simulink model "Week2_Simulation"  (R2024b)
settings: Solver=VariableStepAuto  StartTime=0.0  StopTime=10.0  RelTol=1e-3
undefined symbols (not defined in the file or in its folder): vehicleData
settings Model: Creator=Ian  LastModifiedBy=Ian

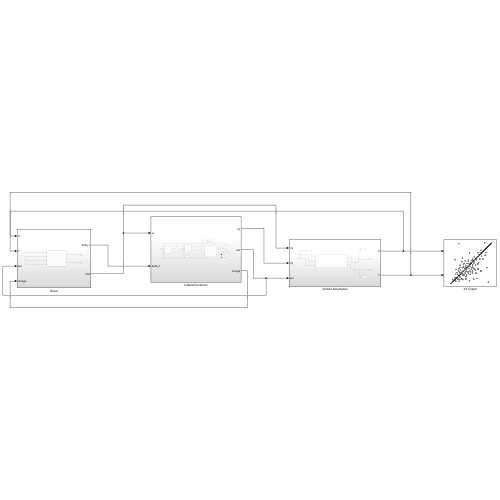
[thumbnail: Simulink's stored preview of the top-level diagram]
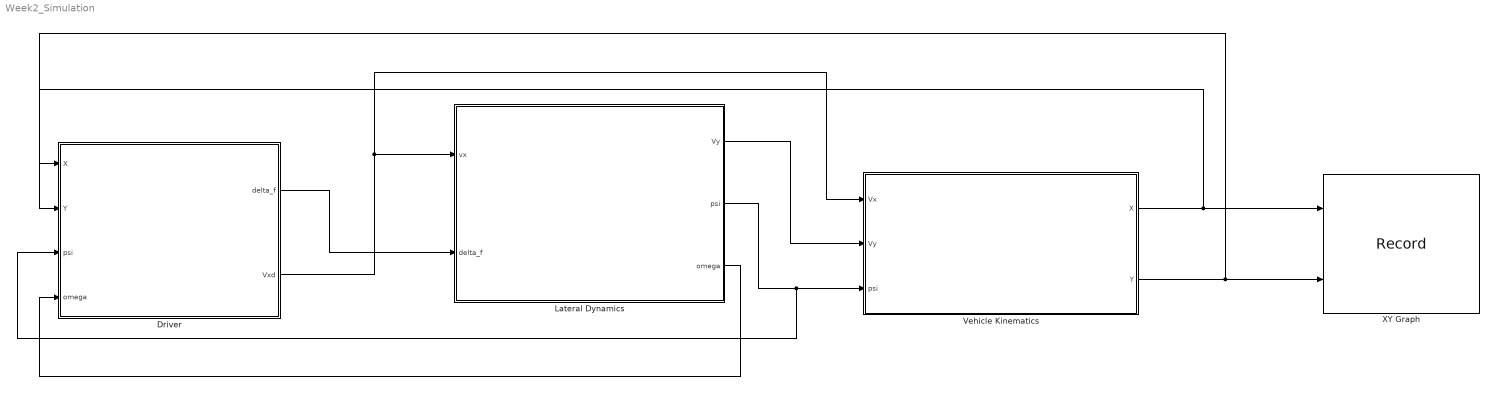
== system Week2_Simulation ==
  Driver : Subsystem
  Lateral Dynamics : Subsystem
  Vehicle Kinematics : Subsystem
  XY Graph : Record  FileSettingsInternal="{\"entries\":[{\"content\":{\"excelSettings\":{\"content\":{},\"type\":\"Streamout.ExcelSettings\"}},\"type\":\"Streamout.FileSettingStorage\",\"uuid\":\"\"}],\"packageUris\":[\"http:\\/\\/schema.mathworks.com\\/mf0\\/streamout_blocks\\/R2020a\"],\"version\":\"1.0\"}"  Layout=[1 1]  SignalsInternal="{\"entries\":[{\"content\":{\"signals\":[{\"content\":{\"blockPath\":[],\"dimensions\":[1],\"domain\":\"\",\"lineColor\":\"#a2142f\",\"plots\":[ 1 ],\"port\":1,\"signalID\":1,\"signalName\":\"XY Graph:1\"},\"type\":\"RecordBlkView.Signal\",\"uuid\":\"\"},{\"content\":{\"blockPath\":[],\"dimensions\":[1],\"domain\":\"\",\"lineColor\":\"#139fff\",\"plots\":[ 1 ],\"port\":2,\"signalID\":2,\"signalName\":\"XY Graph:2\"},\"type\":\"RecordBlkView.Signal\",\"uuid\":\"\"}]},\"type\":\"RecordBlkView.InputSignals\",\"uuid\":\"\"}],\"packageUris\":[\"http:\\/\\/schema.mathworks.com\\/mf0\\/streamout_blocks\\/R2020a\"],\"version\":\"1.0\"}"  VisualizationBindings="{\"xyplotplugin\":{\"info\":[{\"series\":[{\"bindingParametersList\":[{\"parameter\":\"X-Axis\",\"signalID\":1,\"signalName\":\"XY Graph:1\"},{\"parameter\":\"Y-Axis\",\"signalID\":2,\"signalName\":\"XY Graph:2\"}],\"seriesID\":0}],\"subplotID\":1}]}}"  CompatibilityTag=XY
  wires:
  Vehicle Kinematics/2(Y) -> Driver/2(Y), XY Graph/2
  Driver/1(delta_f) -> Lateral Dynamics/2(delta_f)
  Driver/2(Vxd) -> Vehicle Kinematics/1(Vx), Lateral Dynamics/1(vx)
  Vehicle Kinematics/1(X) -> Driver/1(X), XY Graph/1
  Lateral Dynamics/2(psi) -> Driver/3(psi), Vehicle Kinematics/3(psi)
  Lateral Dynamics/1(Vy) -> Vehicle Kinematics/2(Vy)
  Lateral Dynamics/3(omega) -> Driver/4(omega)

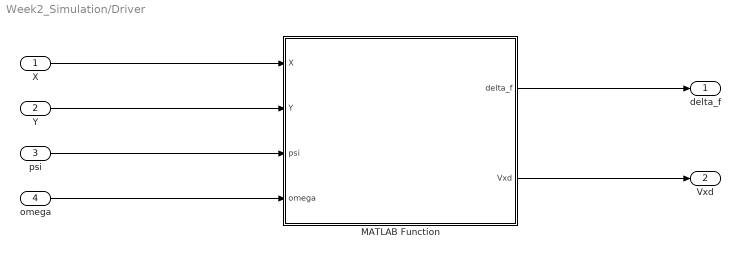
== system Week2_Simulation/Driver ==
  X : Inport
  Y : Inport  Port=2
  psi : Inport  Port=3
  omega : Inport  Port=4
  MATLAB Function : MATLAB Function  TreatAsAtomicUnit=on
  delta_f : Outport
  Vxd : Outport  Port=2
  wires:
  MATLAB Function/2(Vxd) -> Vxd/1
  omega/1 -> MATLAB Function/4(omega)
  X/1 -> MATLAB Function/1(X)
  MATLAB Function/1(delta_f) -> delta_f/1
  psi/1 -> MATLAB Function/3(psi)
  Y/1 -> MATLAB Function/2(Y)

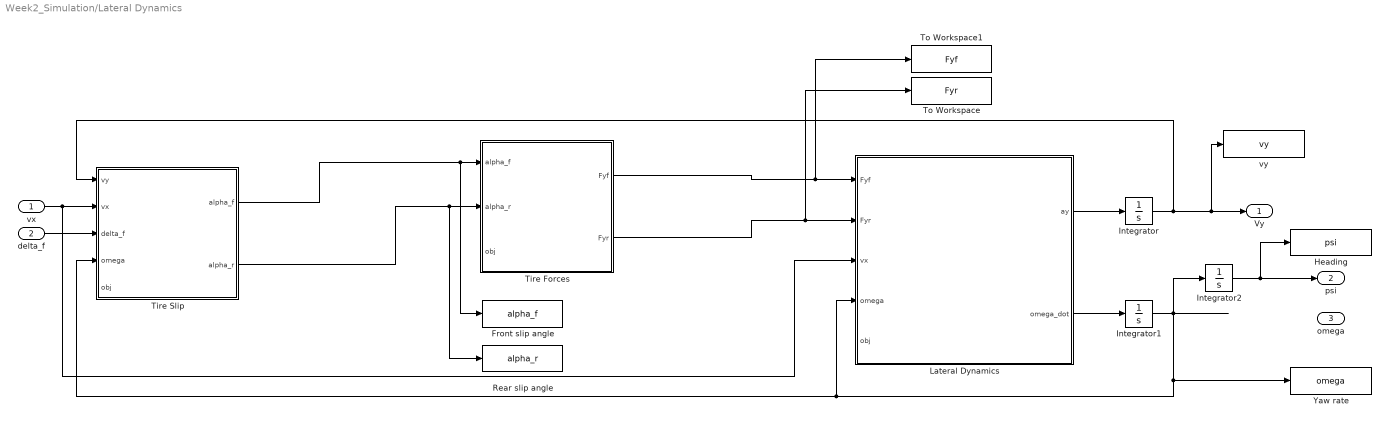
== system Week2_Simulation/Lateral Dynamics ==
  vx : Inport
  delta_f : Inport  Port=2
  Front slip angle : ToWorkspace  VariableName=alpha_f  SaveFormat=Timeseries  SampleTime=-1
  Heading : ToWorkspace  VariableName=psi  SaveFormat=Timeseries  SampleTime=-1
  Integrator : Integrator
  Integrator1 : Integrator
  Integrator2 : Integrator
  Lateral Dynamics : MATLAB Function  TreatAsAtomicUnit=on
  Rear slip angle : ToWorkspace  VariableName=alpha_r  SaveFormat=Timeseries  SampleTime=-1
  Tire Forces : MATLAB Function  TreatAsAtomicUnit=on
  Tire Slip : MATLAB Function  TreatAsAtomicUnit=on
  To Workspace : ToWorkspace  VariableName=Fyr  SaveFormat=Timeseries  SampleTime=-1
  To Workspace1 : ToWorkspace  VariableName=Fyf  SaveFormat=Timeseries  SampleTime=-1
  Yaw rate : ToWorkspace  VariableName=omega  SaveFormat=Timeseries  SampleTime=-1
  vy : ToWorkspace  VariableName=vy  SaveFormat=Timeseries  SampleTime=-1
  Vy : Outport
  psi : Outport  Port=2
  omega : Outport  Port=3
  wires:
  Lateral Dynamics/1(ay) -> Integrator/1
  ? -> Tire Forces/3(obj)
  Integrator2/1 -> psi/1, Heading/1
  vx/1 -> Lateral Dynamics/3(vx), Tire Slip/2(vx)
  Tire Slip/2(alpha_r) -> Rear slip angle/1, Tire Forces/2(alpha_r)
  Tire Forces/1(Fyf) -> To Workspace1/1, Lateral Dynamics/1(Fyf)
  ? -> Lateral Dynamics/5(obj)
  Integrator1/1 -> Yaw rate/1, Tire Slip/4(omega), Lateral Dynamics/4(omega), Integrator2/1
  delta_f/1 -> Tire Slip/3(delta_f)
  Tire Forces/2(Fyr) -> To Workspace/1, Lateral Dynamics/2(Fyr)
  Tire Slip/1(alpha_f) -> Front slip angle/1, Tire Forces/1(alpha_f)
  Integrator/1 -> Vy/1, vy/1, Tire Slip/1(vy)
  Lateral Dynamics/2(omega_dot) -> Integrator1/1
  ? -> Tire Slip/5(obj)

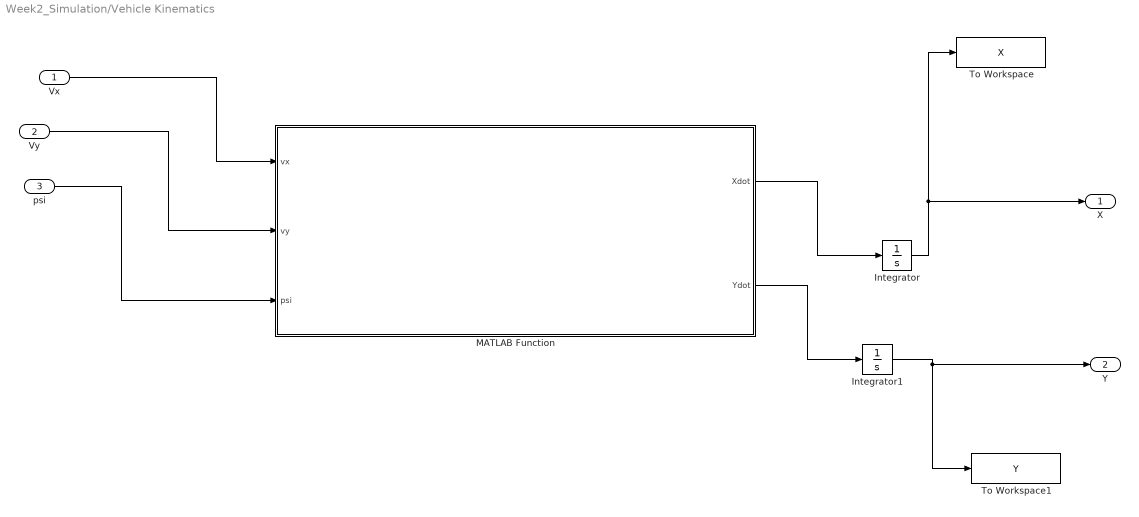
== system Week2_Simulation/Vehicle Kinematics ==
  Vx : Inport
  Vy : Inport  Port=2
  psi : Inport  Port=3
  Integrator : Integrator  InitialCondition=vehicleData.init.X0
  Integrator1 : Integrator  InitialCondition=vehicleData.init.Y0
  MATLAB Function : MATLAB Function  TreatAsAtomicUnit=on
  To Workspace : ToWorkspace  VariableName=X  SaveFormat=Timeseries  SampleTime=-1
  To Workspace1 : ToWorkspace  VariableName=Y  SaveFormat=Timeseries  SampleTime=-1
  X : Outport
  Y : Outport  Port=2
  wires:
  Vx/1 -> MATLAB Function/1(vx)
  MATLAB Function/2(Ydot) -> Integrator1/1
  Integrator/1 -> X/1, To Workspace/1
  Integrator1/1 -> Y/1, To Workspace1/1
  MATLAB Function/1(Xdot) -> Integrator/1
  psi/1 -> MATLAB Function/3(psi)
  Vy/1 -> MATLAB Function/2(vy)

== matlab function Week2_Simulation/Vehicle Kinematics/MATLAB Function ==
  data: Xdot output; Ydot output; vx input; vy input; psi input
function [Xdot, Ydot] = fcn(vx, vy, psi)
    temp = TF(psi) * [vx;vy]; 
    Xdot = temp(1);
    Ydot = temp(2);
end

function y = TF(psi)
    y = [cos(psi), -sin(psi); sin(psi), cos(psi)];
end

== matlab function Week2_Simulation/Driver/MATLAB Function ==
  data: X input; delta_f output; Y input; psi input; omega input; Vxd output
function [delta_f, Vxd] = driver(X, Y, psi, omega)
    
    % Load track data (x_ref, y_ref, psi_ref)
    persistent track_x track_y track_psi;
    if isempty(track_x)
        run('Project2Week2Code.m');
    end

    L = 2.5; 
    Kp = 0.5;  % gain for lateral error; utilizing controller 
    Kd = 0.3;  % gain for heading error
    Kw = 0.1;  % gain for yaw rate damping
    Vmax = 5; % Max speed

    % Find nearest track point
    [~, idx] = min((track_x - X).^2 + (track_y - Y).^2);
    X_ref = track_x(idx);
    Y_ref = track_y(idx);
    psi_ref = track_psi(idx);

    ey = Y - Y_ref;
    epsi = psi - psi_ref;

    delta_f = -Kp * ey - Kd * epsi - Kw * omega;
    
    Vxd = Vmax * (1 - 0.5 * abs(epsi));

    % Bound constraints
    delta_f = max(min(delta_f, 0.5), -0.5);
    Vxd = max(Vxd, 2); 
end

== matlab function Week2_Simulation/Lateral Dynamics/Lateral Dynamics ==
  data: Fyf input; ay output; Fyr input; vx input; omega input; omega_dot output; obj input
function [ay, omega_dot]= fcn(Fyf, Fyr, vx, omega, obj)

Fy = Fyf + Fyr;
ay = Fy/obj.Mass - omega*vx;
M = Fyf*obj.lf - Fyr*obj.lr;
omega_dot = M/obj.Inertia;
end

== matlab function Week2_Simulation/Lateral Dynamics/Tire Forces ==
  data: alpha_f input; Fyf output; alpha_r input; Fyr output; obj input
function [Fyf, Fyr]= fcn(alpha_f, alpha_r, obj)

Fyf = min(obj.Fyfmax, obj.Calpha_f*alpha_f);
Fyr = min(obj.Fyrmax, obj.Calpha_r*alpha_r);
end

== matlab function Week2_Simulation/Lateral Dynamics/Tire Slip ==
  data: vy input; alpha_f output; vx input; delta_f input; omega input; alpha_r output; obj input
function [alpha_f, alpha_r]= fcn(vy, vx, delta_f, omega, obj)

if abs(vx) > obj.vx_threshold1
    alpha_f = delta_f - (vy + omega*obj.lf)/vx;
    alpha_r = -(vy - omega*obj.lr)/vx;
else
    alpha_f = 0;
    alpha_r = 0;
end
end
